simulink model "final_model_pid_height_bueno"  (R2015b)
settings: Solver=ode45  StartTime=0  StopTime=5000  FixedStep=0.001  RelTol=1e-3
libraries: simulink_extras x12, simulink x5, aerolibtransform2 x2, aerolibutil x2, aerolibobsolete x1, aerolibanim x1, aerolibasang x1
(part 2 of 2)

== system final_model_pid_height_bueno/PLANT/Forces and Moments in Take-off/Taxiing2/Aerodynamic Forces /Drag ==
  V : Inport
  S : Inport  Port=2
  rho : Inport  Port=3
  CD0 : Inport  Port=4
  k : Inport  Port=5
  CL : Inport  Port=6
  CD : Subsystem
  Drag : Subsystem
  D : Outport
  wires:
  V/1 -> Drag/1(V)
  rho/1 -> Drag/3(rho)
  S/1 -> Drag/2(S)
  Drag/1(D) -> D/1
  CD/1(CD) -> Drag/4(CD)
  CL/1 -> CD/3(CL)
  CD0/1 -> CD/1(CD0)
  k/1 -> CD/2(k)

== system final_model_pid_height_bueno/PLANT/Forces and Moments in Take-off/Taxiing2/Aerodynamic Forces /F Normales ==
  mu_r : Inport
  N2 : Inport  Port=2
  Product1 : Product
  Fr2 : Outport
  wires:
  mu_r/1 -> Product1/1
  N2/1 -> Product1/2
  Product1/1 -> Fr2/1

== system final_model_pid_height_bueno/PLANT/Forces and Moments in Take-off/Taxiing2/Aerodynamic Forces /Fx equation ==
  T : Inport
  D : Inport  Port=2
  Fr2 : Inport  Port=3
  Add2 : Sum  Inputs=+++
  Gain : Gain  Gain=-1
  Gain2 : Gain  Gain=-1
  Fx : Outport
  wires:
  Fr2/1 -> Gain2/1
  Add2/1 -> Fx/1
  Gain/1 -> Add2/2
  D/1 -> Gain/1
  Gain2/1 -> Add2/3
  T/1 -> Add2/1

== system final_model_pid_height_bueno/PLANT/Forces and Moments in Take-off/Taxiing2/Aerodynamic Forces /Fz = 0 ==
  L : Inport
  W : Inport  Port=2
  T : Inport  Port=3
  Add1 : Sum  Inputs=+--
  Scope : Scope
  N2 : Outport
  wires:
  Add1/1 -> N2/1
  L/1 -> Scope/1, Add1/2
  W/1 -> Add1/1
  T/1 -> Add1/3

== system final_model_pid_height_bueno/PLANT/Forces and Moments in Take-off/Taxiing2/Aerodynamic Forces /Lift ==
  V : Inport
  S : Inport  Port=2
  rho : Inport  Port=3
  alpha : Inport  Port=4
  CL0 : Inport  Port=5
  CL_alpha : Inport  Port=6
  "CL " : Subsystem
  Lift : Subsystem
  CL : Outport
  L : Outport  Port=2
  wires:
  rho/1 -> Lift/3(rho)
  S/1 -> Lift/2(S)
  V/1 -> Lift/1(V)
  "CL "/1("CL ") -> CL/1, Lift/4(CL)
  CL0/1 -> "CL "/1(CL0)
  CL_alpha/1 -> "CL "/2(CL_alpha)
  alpha/1 -> "CL "/3(alpha)
  Lift/1(L) -> L/1

== system final_model_pid_height_bueno/PLANT/Forces and Moments in Take-off/Taxiing2/Aerodynamic Moments / My ==
  delta_e : Inport
  rho_0 : Inport  Port=2
  S : Inport  Port=3
  c : Inport  Port=4
  x2 : Inport  Port=5
  Fr2 : Inport  Port=6
  zg : Inport  Port=7
  N2 : Inport  Port=8
  V : Inport  Port=9
  alpha : Inport  Port=10
  theta' : Inport  Port=11
  Add1 : Sum  Inputs=+--
  CM_A : Subsystem
  MA : Subsystem
  Product : Product
  Product1 : Product
  My : Outport
  wires:
  CM_A/1(CM_A) -> MA/4(CM_A)
  delta_e/1 -> CM_A/2(delta)
  c/1 -> MA/5(c)
  MA/1(MA) -> Add1/1
  zg/1 -> Product/2
  x2/1 -> Product1/1
  Product/1 -> Add1/2
  Product1/1 -> Add1/3
  Add1/1 -> My/1
  N2/1 -> Product1/2
  theta'/1 -> CM_A/3(theta')
  alpha/1 -> CM_A/1(alpha)
  Fr2/1 -> Product/1
  V/1 -> MA/1(V)
  S/1 -> MA/2(S)
  rho_0/1 -> MA/3(rho_0)

== system final_model_pid_height_bueno/PLANT/Forces and Moments in Take-off/Transition/Aerodynamic Forces /Drag ==
  V : Inport
  S : Inport  Port=2
  rho : Inport  Port=3
  CD0 : Inport  Port=4
  k : Inport  Port=5
  CL : Inport  Port=6
  CD : Subsystem
  Drag : Subsystem
  D : Outport
  wires:
  V/1 -> Drag/1(V)
  rho/1 -> Drag/3(rho)
  S/1 -> Drag/2(S)
  Drag/1(D) -> D/1
  CD/1(CD) -> Drag/4(CD)
  CL/1 -> CD/3(CL)
  CD0/1 -> CD/1(CD0)
  k/1 -> CD/2(k)

== system final_model_pid_height_bueno/PLANT/Forces and Moments in Take-off/Transition/Aerodynamic Forces /Fx equation ==
  Tx : Inport
  D : Inport  Port=2
  Wx : Inport  Port=3
  Add2 : Sum  Inputs=+++
  Gain : Gain  Gain=-1
  Fx : Outport
  wires:
  Add2/1 -> Fx/1
  Tx/1 -> Add2/1
  Gain/1 -> Add2/2
  D/1 -> Gain/1
  Wx/1 -> Add2/3

== system final_model_pid_height_bueno/PLANT/Forces and Moments in Take-off/Transition/Aerodynamic Forces /Fy equation ==
  V : Inport
  "rho " : Inport  Port=2
  S : Inport  Port=3
  "beta " : Inport  Port=4
  delta_a : Inport  Port=5
  delta_r : Inport  Port=6
  "Dynamic pressure " : Subsystem
  Lateral Force Coefficient : Subsystem
  Product : Product  Inputs=3
  Fy : Outport
  wires:
  V/1 -> "Dynamic pressure "/1(V)
  "rho "/1 -> "Dynamic pressure "/2("rho ")
  "Dynamic pressure "/1(q) -> Product/1
  S/1 -> Product/2
  Product/1 -> Fy/1
  "beta "/1 -> Lateral Force Coefficient/1("beta ")
  Lateral Force Coefficient/1(C_Y) -> Product/3
  delta_a/1 -> Lateral Force Coefficient/2(delta_a)
  delta_r/1 -> Lateral Force Coefficient/3(delta_r)

== system final_model_pid_height_bueno/PLANT/Forces and Moments in Take-off/Transition/Aerodynamic Forces /Fz Equation  ==
  L : Inport
  "Wz " : Inport  Port=2
  Tz : Inport  Port=3
  Add1 : Sum  Inputs=+-+
  Scope1 : Scope
  Scope2 : Scope
  Fz : Outport
  wires:
  Add1/1 -> Fz/1
  L/1 -> Add1/2
  Tz/1 -> Scope1/1, Add1/3
  "Wz "/1 -> Scope2/1, Add1/1

== system final_model_pid_height_bueno/PLANT/Forces and Moments in Take-off/Transition/Aerodynamic Forces /Lift ==
  V : Inport
  S : Inport  Port=2
  rho : Inport  Port=3
  alpha : Inport  Port=4
  CL0 : Inport  Port=5
  CL_alpha : Inport  Port=6
  "CL " : Subsystem
  Lift : Subsystem
  CL : Outport
  L : Outport  Port=2
  wires:
  rho/1 -> Lift/3(rho)
  S/1 -> Lift/2(S)
  V/1 -> Lift/1(V)
  "CL "/1("CL ") -> CL/1, Lift/4(CL)
  CL0/1 -> "CL "/1(CL0)
  CL_alpha/1 -> "CL "/2(CL_alpha)
  alpha/1 -> "CL "/3(alpha)
  Lift/1(L) -> L/1

== system final_model_pid_height_bueno/PLANT/Forces and Moments in Take-off/Transition/Aerodynamic Moments /Pitch Moment ==
  alpha : Inport
  delta_e : Inport  Port=2
  V : Inport  Port=3
  rho : Inport  Port=4
  S : Inport  Port=5
  c : Inport  Port=6
  theta' : Inport  Port=7
  C_mA : Subsystem
  Pitch Moment : Subsystem
  Scope : Scope
  "M_A " : Outport
  wires:
  alpha/1 -> C_mA/1(alpha)  "1"
  V/1 -> Pitch Moment/2(V)
  rho/1 -> Pitch Moment/3(rho)
  S/1 -> Pitch Moment/4(S)
  delta_e/1 -> C_mA/2(delta_e)
  c/1 -> Pitch Moment/5(c)
  theta'/1 -> C_mA/3(theta')
  Pitch Moment/1(M_A) -> "M_A "/1
  C_mA/1(C_mA) -> Scope/1, Pitch Moment/1(C_mA)

== system final_model_pid_height_bueno/PLANT/Forces and Moments in Take-off/Transition/Aerodynamic Moments /Roll Moment ==
  b : Inport
  "beta " : Inport  Port=2
  delta_a : Inport  Port=3
  delta_r : Inport  Port=4
  S : Inport  Port=5
  "rho " : Inport  Port=6
  V : Inport  Port=7
  "Dynamic pressure " : Subsystem
  Product : Product  Inputs=4
  Roll Moment Coefficient : Subsystem
  L_A : Outport
  wires:
  V/1 -> "Dynamic pressure "/1(V)
  "rho "/1 -> "Dynamic pressure "/2("rho ")
  "Dynamic pressure "/1(q) -> Product/1
  S/1 -> Product/2
  Product/1 -> L_A/1
  "beta "/1 -> Roll Moment Coefficient/1("beta ")
  Roll Moment Coefficient/1(C_l) -> Product/4
  delta_a/1 -> Roll Moment Coefficient/2(delta_a)
  delta_r/1 -> Roll Moment Coefficient/3(delta_r)
  b/1 -> Product/3

== system final_model_pid_height_bueno/PLANT/Forces and Moments in Take-off/Transition/Aerodynamic Moments /Yaw Moment ==
  S : Inport
  "rho " : Inport  Port=2
  V : Inport  Port=3
  delta_r : Inport  Port=4
  delta_a : Inport  Port=5
  "beta " : Inport  Port=6
  b : Inport  Port=7
  "Dynamic pressure " : Subsystem
  Product : Product  Inputs=4
  Yaw Moment Coefficient : Subsystem
  N_A : Outport
  wires:
  V/1 -> "Dynamic pressure "/1(V)
  "rho "/1 -> "Dynamic pressure "/2("rho ")
  "Dynamic pressure "/1(q) -> Product/1
  S/1 -> Product/2
  Product/1 -> N_A/1
  "beta "/1 -> Yaw Moment Coefficient/1("beta ")
  Yaw Moment Coefficient/1(C_n) -> Product/4
  delta_a/1 -> Yaw Moment Coefficient/2(delta_a)
  delta_r/1 -> Yaw Moment Coefficient/3(delta_r)
  b/1 -> Product/3

== system final_model_pid_height_bueno/PLANT/Forces and Moments in Take-off/Taxiing/Aerodynamic Forces /Drag/CD ==
  CD0 : Inport
  k : Inport  Port=2
  CL : Inport  Port=3
  Add : Sum
  Product : Product  Inputs=3
  CD : Outport
  wires:
  CD0/1 -> Add/1
  Product/1 -> Add/2
  k/1 -> Product/1
  Add/1 -> CD/1
  CL/1 -> Product/3, Product/2

== system final_model_pid_height_bueno/PLANT/Forces and Moments in Take-off/Taxiing/Aerodynamic Forces /Drag/Drag ==
  V : Inport
  S : Inport  Port=2
  rho : Inport  Port=3
  CD : Inport  Port=4
  "0.5 " : Constant  Value=0.5
  Product : Product  Inputs=6
  D : Outport
  wires:
  rho/1 -> Product/2
  V/1 -> Product/4, Product/5
  CD/1 -> Product/6
  Product/1 -> D/1
  S/1 -> Product/3
  "0.5 "/1 -> Product/1

== system final_model_pid_height_bueno/PLANT/Forces and Moments in Take-off/Taxiing/Aerodynamic Forces /Lift/CL  ==
  CL0 : Inport
  CL_alpha : Inport  Port=2
  alpha : Inport  Port=3
  Add : Sum
  Product : Product
  "CL " : Outport
  wires:
  CL0/1 -> Add/1
  CL_alpha/1 -> Product/1
  Product/1 -> Add/2
  alpha/1 -> Product/2
  Add/1 -> "CL "/1

== system final_model_pid_height_bueno/PLANT/Forces and Moments in Take-off/Taxiing/Aerodynamic Forces /Lift/Lift ==
  V : Inport
  S : Inport  Port=2
  rho : Inport  Port=3
  CL : Inport  Port=4
  "0.5 " : Constant  Value=0.5
  Product : Product  Inputs=6
  L : Outport
  wires:
  rho/1 -> Product/2
  V/1 -> Product/4, Product/5
  CL/1 -> Product/6
  Product/1 -> L/1
  S/1 -> Product/3
  "0.5 "/1 -> Product/1

== system final_model_pid_height_bueno/PLANT/Forces and Moments in Take-off/Taxiing/Aerodynamic Moments /My /CM_A ==
  alpha : Inport
  delta : Inport  Port=2
  Add : Sum  Inputs=+++
  Cm0 : Constant  Value=0.04
  Cm_alpha : Constant  Value=-0.65
  Cm_delta : Constant  Value=-1.369
  Product : Product
  Product1 : Product
  CM_A : Outport
  wires:
  alpha/1 -> Product/1
  Cm_alpha/1 -> Product/2
  Cm0/1 -> Add/1
  delta/1 -> Product1/2
  Cm_delta/1 -> Product1/1
  Add/1 -> CM_A/1
  Product1/1 -> Add/3
  Product/1 -> Add/2

== system final_model_pid_height_bueno/PLANT/Forces and Moments in Take-off/Taxiing/Aerodynamic Moments /My /MA ==
  V : Inport
  S : Inport  Port=2
  rho : Inport  Port=3
  CM_A : Inport  Port=4
  c : Inport  Port=5
  "0.5 " : Constant  Value=0.5
  Product : Product  Inputs=7
  MA : Outport
  wires:
  c/1 -> Product/6
  "0.5 "/1 -> Product/1
  S/1 -> Product/3
  Product/1 -> MA/1
  CM_A/1 -> Product/7
  V/1 -> Product/5, Product/4
  rho/1 -> Product/2

== system final_model_pid_height_bueno/PLANT/Forces and Moments in Take-off/Taxiing2/Aerodynamic Forces /Drag/CD ==
  CD0 : Inport
  k : Inport  Port=2
  CL : Inport  Port=3
  Add : Sum
  Product : Product  Inputs=3
  CD : Outport
  wires:
  CD0/1 -> Add/1
  Product/1 -> Add/2
  k/1 -> Product/1
  Add/1 -> CD/1
  CL/1 -> Product/3, Product/2

== system final_model_pid_height_bueno/PLANT/Forces and Moments in Take-off/Taxiing2/Aerodynamic Forces /Drag/Drag ==
  V : Inport
  S : Inport  Port=2
  rho : Inport  Port=3
  CD : Inport  Port=4
  "0.5 " : Constant  Value=0.5
  Product : Product  Inputs=6
  D : Outport
  wires:
  rho/1 -> Product/2
  V/1 -> Product/4, Product/5
  CD/1 -> Product/6
  Product/1 -> D/1
  S/1 -> Product/3
  "0.5 "/1 -> Product/1

== system final_model_pid_height_bueno/PLANT/Forces and Moments in Take-off/Taxiing2/Aerodynamic Forces /Lift/CL  ==
  CL0 : Inport
  CL_alpha : Inport  Port=2
  alpha : Inport  Port=3
  Add : Sum
  Product : Product
  "CL " : Outport
  wires:
  CL0/1 -> Add/1
  CL_alpha/1 -> Product/1
  Product/1 -> Add/2
  alpha/1 -> Product/2
  Add/1 -> "CL "/1

== system final_model_pid_height_bueno/PLANT/Forces and Moments in Take-off/Taxiing2/Aerodynamic Forces /Lift/Lift ==
  V : Inport
  S : Inport  Port=2
  rho : Inport  Port=3
  CL : Inport  Port=4
  "0.5 " : Constant  Value=0.5
  Product : Product  Inputs=6
  L : Outport
  wires:
  rho/1 -> Product/2
  V/1 -> Product/4, Product/5
  CL/1 -> Product/6
  Product/1 -> L/1
  S/1 -> Product/3
  "0.5 "/1 -> Product/1

== system final_model_pid_height_bueno/PLANT/Forces and Moments in Take-off/Taxiing2/Aerodynamic Moments / My/CM_A ==
  alpha : Inport
  delta : Inport  Port=2
  theta' : Inport  Port=3
  Add : Sum  Inputs=++++
  Cm0 : Constant  Value=0.04
  Cm_alpha : Constant  Value=-0.65
  Cm_delta : Constant  Value=-1.369
  Cm_q : Constant  Value=-15.20
  Product : Product
  Product1 : Product
  Product2 : Product
  CM_A : Outport
  wires:
  Product/1 -> Add/2
  Product1/1 -> Add/3
  Add/1 -> CM_A/1
  Cm_delta/1 -> Product1/1
  delta/1 -> Product1/2
  Cm0/1 -> Add/1
  Cm_alpha/1 -> Product/2
  alpha/1 -> Product/1
  Cm_q/1 -> Product2/1
  theta'/1 -> Product2/2
  Product2/1 -> Add/4

== system final_model_pid_height_bueno/PLANT/Forces and Moments in Take-off/Taxiing2/Aerodynamic Moments / My/MA ==
  V : Inport
  S : Inport  Port=2
  rho_0 : Inport  Port=3
  CM_A : Inport  Port=4
  c : Inport  Port=5
  "0.5 " : Constant  Value=0.5
  Product : Product  Inputs=7
  MA : Outport
  wires:
  rho_0/1 -> Product/2
  V/1 -> Product/5, Product/4
  CM_A/1 -> Product/7
  Product/1 -> MA/1
  S/1 -> Product/3
  "0.5 "/1 -> Product/1
  c/1 -> Product/6

== system final_model_pid_height_bueno/PLANT/Forces and Moments in Take-off/Transition/Aerodynamic Forces /Drag/CD ==
  CD0 : Inport
  k : Inport  Port=2
  CL : Inport  Port=3
  Add : Sum
  Product : Product  Inputs=3
  CD : Outport
  wires:
  CD0/1 -> Add/1
  Product/1 -> Add/2
  k/1 -> Product/1
  Add/1 -> CD/1
  CL/1 -> Product/3, Product/2

== system final_model_pid_height_bueno/PLANT/Forces and Moments in Take-off/Transition/Aerodynamic Forces /Drag/Drag ==
  V : Inport
  S : Inport  Port=2
  rho : Inport  Port=3
  CD : Inport  Port=4
  "0.5 " : Constant  Value=0.5
  Product : Product  Inputs=6
  D : Outport
  wires:
  rho/1 -> Product/2
  V/1 -> Product/4, Product/5
  CD/1 -> Product/6
  Product/1 -> D/1
  S/1 -> Product/3
  "0.5 "/1 -> Product/1

== system final_model_pid_height_bueno/PLANT/Forces and Moments in Take-off/Transition/Aerodynamic Forces /Fy equation/Dynamic pressure  ==
  V : Inport
  "rho " : Inport  Port=2
  Constant : Constant  Value=0.5
  Math Function : Math  Operator=square  SaturateOnIntegerOverflow=on
  Product : Product  Inputs=3
  q : Outport
  wires:
  Math Function/1 -> Product/1
  "rho "/1 -> Product/3
  Product/1 -> q/1
  Constant/1 -> Product/2
  V/1 -> Math Function/1

== system final_model_pid_height_bueno/PLANT/Forces and Moments in Take-off/Transition/Aerodynamic Forces /Fy equation/Lateral Force Coefficient ==
  "beta " : Inport
  delta_a : Inport  Port=2
  delta_r : Inport  Port=3
  C_Y0 : Constant  Value=0
  C_Ybeta : Constant  Value=-0.404
  C_Ydelta_a : Constant  Value=0
  C_Ydelta_r : Constant  Value=0.187
  Product1 : Product
  Product2 : Product
  Product3 : Product
  "Sum " : Sum  Inputs=++++
  C_Y : Outport
  wires:
  "beta "/1 -> Product1/1
  C_Ybeta/1 -> Product1/2
  delta_a/1 -> Product2/1
  C_Ydelta_a/1 -> Product2/2
  delta_r/1 -> Product3/1
  C_Ydelta_r/1 -> Product3/2
  C_Y0/1 -> "Sum "/1
  Product1/1 -> "Sum "/2
  Product2/1 -> "Sum "/3
  Product3/1 -> "Sum "/4
  "Sum "/1 -> C_Y/1

== system final_model_pid_height_bueno/PLANT/Forces and Moments in Take-off/Transition/Aerodynamic Forces /Lift/CL  ==
  CL0 : Inport
  CL_alpha : Inport  Port=2
  alpha : Inport  Port=3
  Add : Sum
  Product : Product
  "CL " : Outport
  wires:
  CL0/1 -> Add/1
  CL_alpha/1 -> Product/1
  Product/1 -> Add/2
  alpha/1 -> Product/2
  Add/1 -> "CL "/1

== system final_model_pid_height_bueno/PLANT/Forces and Moments in Take-off/Transition/Aerodynamic Forces /Lift/Lift ==
  V : Inport
  S : Inport  Port=2
  rho : Inport  Port=3
  CL : Inport  Port=4
  "0.5 " : Constant  Value=0.5
  Product : Product  Inputs=6
  L : Outport
  wires:
  rho/1 -> Product/2
  V/1 -> Product/4, Product/5
  CL/1 -> Product/6
  Product/1 -> L/1
  S/1 -> Product/3
  "0.5 "/1 -> Product/1

== system final_model_pid_height_bueno/PLANT/Forces and Moments in Take-off/Transition/Aerodynamic Moments /Pitch Moment/C_mA ==
  alpha : Inport
  delta_e : Inport  Port=2
  theta' : Inport  Port=3
  Add : Sum  Inputs=++++
  C_m0 : Constant  Value=0.04
  C_malpha : Constant  Value=-0.65
  C_mdelta_e : Constant  Value=-1.369
  C_mq : Constant  Value=-15.20
  Product : Product
  Product1 : Product
  Product2 : Product
  C_mA : Outport
  wires:
  Product/1 -> Add/2
  Product1/1 -> Add/3
  Add/1 -> C_mA/1
  C_mdelta_e/1 -> Product1/1
  delta_e/1 -> Product1/2
  C_m0/1 -> Add/1
  C_malpha/1 -> Product/2
  alpha/1 -> Product/1
  C_mq/1 -> Product2/1
  theta'/1 -> Product2/2
  Product2/1 -> Add/4

== system final_model_pid_height_bueno/PLANT/Forces and Moments in Take-off/Transition/Aerodynamic Moments /Pitch Moment/Pitch Moment ==
  C_mA : Inport
  V : Inport  Port=2
  rho : Inport  Port=3
  S : Inport  Port=4
  c : Inport  Port=5
  "0.5 " : Constant  Value=0.5
  Product : Product  Inputs=7
  M_A : Outport
  wires:
  rho/1 -> Product/2
  V/1 -> Product/4, Product/5
  C_mA/1 -> Product/7
  Product/1 -> M_A/1
  S/1 -> Product/3
  "0.5 "/1 -> Product/1
  c/1 -> Product/6

== system final_model_pid_height_bueno/PLANT/Forces and Moments in Take-off/Transition/Aerodynamic Moments /Roll Moment/Dynamic pressure  ==
  V : Inport
  "rho " : Inport  Port=2
  Constant : Constant  Value=0.5
  Math Function : Math  Operator=square  SaturateOnIntegerOverflow=on
  Product : Product  Inputs=3
  q : Outport
  wires:
  Math Function/1 -> Product/1
  "rho "/1 -> Product/3
  Product/1 -> q/1
  Constant/1 -> Product/2
  V/1 -> Math Function/1

== system final_model_pid_height_bueno/PLANT/Forces and Moments in Take-off/Transition/Aerodynamic Moments /Roll Moment/Roll Moment Coefficient ==
  "beta " : Inport
  delta_a : Inport  Port=2
  delta_r : Inport  Port=3
  C_l0 : Constant  Value=0
  C_lbeta : Constant  Value=-0.0895
  C_ldelta_a : Constant  Value=0.2290
  C_ldelta_r : Constant  Value=0.0147
  Product1 : Product
  Product2 : Product
  Product3 : Product
  "Sum " : Sum  Inputs=++++
  C_l : Outport
  wires:
  "beta "/1 -> Product1/1
  C_lbeta/1 -> Product1/2
  delta_a/1 -> Product2/1
  C_ldelta_a/1 -> Product2/2
  delta_r/1 -> Product3/1
  C_ldelta_r/1 -> Product3/2
  C_l0/1 -> "Sum "/1
  Product1/1 -> "Sum "/2
  Product2/1 -> "Sum "/3
  Product3/1 -> "Sum "/4
  "Sum "/1 -> C_l/1

== system final_model_pid_height_bueno/PLANT/Forces and Moments in Take-off/Transition/Aerodynamic Moments /Yaw Moment/Dynamic pressure  ==
  V : Inport
  "rho " : Inport  Port=2
  Constant : Constant  Value=0.5
  Math Function : Math  Operator=square  SaturateOnIntegerOverflow=on
  Product : Product  Inputs=3
  q : Outport
  wires:
  Math Function/1 -> Product/1
  "rho "/1 -> Product/3
  Product/1 -> q/1
  Constant/1 -> Product/2
  V/1 -> Math Function/1

== system final_model_pid_height_bueno/PLANT/Forces and Moments in Take-off/Transition/Aerodynamic Moments /Yaw Moment/Yaw Moment Coefficient ==
  "beta " : Inport
  delta_a : Inport  Port=2
  delta_r : Inport  Port=3
  C_n0 : Constant  Value=0
  C_nbeta : Constant  Value=0.0907
  C_ndelta_a : Constant  Value=-0.0504
  C_ndelta_r : Constant  Value=-0.0805
  Product1 : Product
  Product2 : Product
  Product3 : Product
  "Sum " : Sum  Inputs=++++
  C_n : Outport
  wires:
  "beta "/1 -> Product1/1
  C_nbeta/1 -> Product1/2
  delta_a/1 -> Product2/1
  C_ndelta_a/1 -> Product2/2
  delta_r/1 -> Product3/1
  C_ndelta_r/1 -> Product3/2
  C_n0/1 -> "Sum "/1
  Product1/1 -> "Sum "/2
  Product2/1 -> "Sum "/3
  Product3/1 -> "Sum "/4
  "Sum "/1 -> C_n/1

== matlab function final_model_pid_height_bueno/AUTOPILOT/Theta control/THETA HIGH HEIGHTS ==
  data: theta_d output; h input; h_d input; theta_descenso input
function theta_d = fcn(h,h_d,theta_descenso)
%#codegen

if h_d + h >= 4
    theta_d = ((h_d + h)/1750) + ((h_d)/4500) - (1/4.5) + 4;
elseif h_d + h < 4
    theta_d = theta_descenso;
else
    theta_d = theta_descenso;
end

== matlab function final_model_pid_height_bueno/AUTOPILOT/Theta control/THETA SWITCH ==
  data: theta_d output; a input; h_d input; b input
function theta_d = fcn(a,h_d,b)
%#codegen

if h_d <= 3000
    theta_d = a;
else
    theta_d = b;
end

== matlab function final_model_pid_height_bueno/AUTOPILOT/Theta control/THETA LOW HEIGHTS ==
  data: theta_d output; h input; h_d input; theta_descenso input
function theta_d = fcn(h,h_d,theta_descenso)
%#codegen

if h_d + h >= 4
    theta_d = ((h_d + h)/1750) + ((h_d)/4500) - (1/4.5) + 2.5;
elseif h_d + h < 4
    theta_d = theta_descenso;
else
    theta_d = theta_descenso;
end

== matlab function final_model_pid_height_bueno/AUTOPILOT/PHI ==
  data: x input; phi2 input; desired_phi output; phi1 input; threshold input
function desired_phi = fcn(x,phi2,phi1,threshold)
%#codegen

if x >= threshold
    desired_phi = phi2;
else
    desired_phi = phi1;
end

== matlab function final_model_pid_height_bueno/AUTOPILOT/THETA//HEIGHT SWITCH ==
  data: h_controller input; delta_e output; h input; h_d input; theta_controller input
function delta_e = fcn(h_controller,h,h_d,theta_controller)
%#codegen

if h_d - h >= 4
    delta_e = theta_controller;
elseif h_d - h < 4
    delta_e = theta_controller;
else
    delta_e = h_controller;
end

== matlab function final_model_pid_height_bueno/AUTOPILOT/YAW ==
  data: x input; psi2 input; desired_psi output; psi1 input; threshold input
function desired_psi = fcn(x,psi2,psi1,threshold)
%#codegen

if x >= threshold
    desired_psi = psi2;
else
    desired_psi = psi1;
end
